simulink model "GUAM"  (R2024a)
settings: Solver=FixedStepAuto  StartTime=0.0  StopTime=SimIn.stopTime  FixedStep=0.01  RelTol=1e-6
InitFcn:
  | S = 0;
values from neighbouring files (symbols this model uses):
  SimIn = setup(SimIn, target)    [simSetup.m]
undefined symbols (not defined in the file or in its folder): SimPar
libraries: simulink x6, eeGeneralControl x5, dspstat3 x5, aerolibfltsims x2, dspnetwork x2
settings Model: SnapshotBufferSize=20  SnapshotInterval=1  PacingRate=0.100000  Creator=tbritton  LastModifiedBy=azmol
settings SolverCC: AlgebraicLoopSolver=TrustRegion  AutoInsertRateTranBlk=on  InsertRTBMode=Never (minimum delay)
settings DataIOCC: SaveFormat=StructureWithTime  SaveOutput=off  DSMLogging=off  SaveTime=off  ReturnWorkspaceOutputs=off
settings OptimizationCC: ReuseModelBlockBuffer=off
settings DebuggingCC: ReadBeforeWriteMsg=DisableAll  WriteAfterWriteMsg=DisableAll  WriteAfterReadMsg=DisableAll  UnconnectedInputMsg=warning  UnconnectedOutputMsg=warning  UnconnectedLineMsg=warning  InitInArrayFormatMsg=none
settings ModelReferenceCC: UpdateModelReferenceTargets=IfOutOfDate  EnableRefExpFcnMdlSchedulingChecks=on
settings SFSimCC: SFSimEcho=off  CustomCodeUndefinedFunction=UseInterfaceOnly
settings RTWCC: GPUComputeCapability=3.5  DLArmComputeVersion=19.05

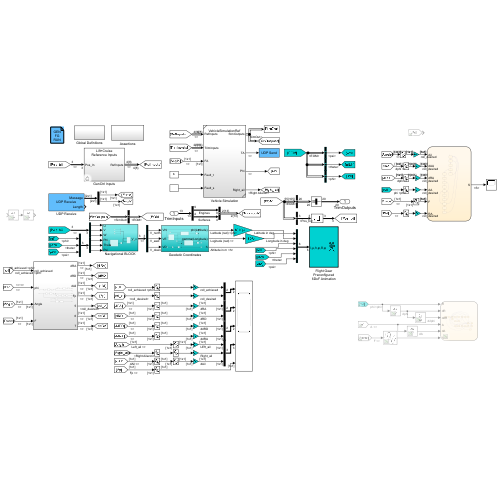
[thumbnail: Simulink's stored preview of the top-level diagram]
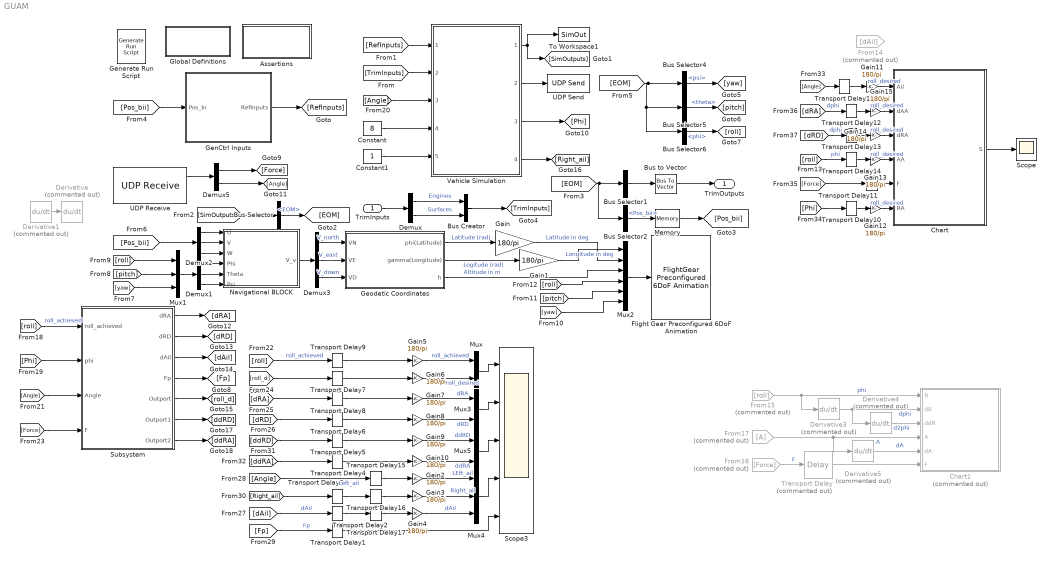
== system GUAM ==
  TrimInputs : Inport
  Assertions : Subsystem
  Bus Creator : BusCreator  Inputs=2  OutDataTypeStr=Bus: BUS_TRIM_INPUT
  Bus Selector : BusSelector  OutputSignals=Vehicle.EOM
  Bus Selector1 : BusSelector  OutputSignals=AirRelativeData.Veas,AirRelativeData.Vtot,AirRelativeData.alpha,AirRelativeData.beta,WorldRelativeData.gamma,WorldRelativeData.chi,InertialData.Asensed_bIb,AirRelativeData.Vtotdot,AirRelativeData.alphadot,AirRelativeData.betadot,WorldRelativeData.gammadot,WorldRelativeData.chidot,WorldRelativeData.VelDtH_bEh,WorldRelativeData.Euler.phi,WorldRelativeData.Euler.theta,WorldRelativeData.Euler.psi  OutputAsBus=on
  Bus Selector2 : BusSelector  OutputSignals=InertialData.Pos_bii
  Bus Selector4 : BusSelector  OutputSignals=WorldRelativeData.Euler.psi
  Bus Selector5 : BusSelector  OutputSignals=WorldRelativeData.Euler.theta
  Bus Selector6 : BusSelector  OutputSignals=WorldRelativeData.Euler.phi
  Bus to Vector : BusToVector
  Chart : Stateflow chart  TreatAsAtomicUnit=on
  Chart1 : Stateflow chart  Commented=on  TreatAsAtomicUnit=on
      settings: PortSchema="{\"entries\":[{\"content\":{\"sides\":[{\"content\":{\"connectorIds\":[\"In6\",\"In3\",\"In2\",\"In4\",\"In1\",\"In5\"]},\"type\":\"ConnectorPlacement.EquallySpacedRectSide\",\"uuid\":\"2c3cc659-f24d-4f43-a956-b726e491f665\"},{\"content\":{\"side\":\"RIGHT\"},\"type\":\"ConnectorPlacement.EquallySpacedRectSide\",\"uuid\":\"d5ffd018-8575-4a45-b274-c52cea02283c\"},{\"content\":{\"side\":\"TOP\"},\"type\":\"ConnectorPlacement.EquallySpacedRectSide\",\"uuid\":\"e163f1a1-9c0c-475f-9ea7-59fb8c09f8a6\"}]},\"type\":\"ConnectorPlacement.EquallySpacedConnector\",\"uuid\":\"e013bf2e-a49f-4647-8efb-e6a80c4823c8\"}],\"packageUris\":[\"http://schema.mathworks.com/mf0/Connector/R2020b\"],\"version\":\"1.0\"}"
  Constant : Constant  Value=8
  Constant1 : Constant
  Demux : Demux  Outputs=[SimIn.Trim.numEngines SimIn.Trim.numSurfaces]
  Demux1 : Demux  Outputs=3
  Demux2 : Demux  Outputs=3
  Demux3 : Demux  Outputs=3
  Demux5 : Demux  Outputs=2
  Derivative{,1,3..5} (5 alike) : Derivative  Commented=on
  Flight Gear Preconfigured 6DoF Animation : aerolibfltsims/FlightGear Preconfigured 6DoF Animation  xFlightGearVersion=v2019.1  DestinationIpAddress=127.0.0.1  DestinationPort=5502  SampleTime=1/100  packetVersion=24
  From14 : From  Commented=on  GotoTag=dAil
  From15 : From  Commented=on  GotoTag=roll
  From16 : From  Commented=on  GotoTag=Force
  From17 : From  Commented=on
  Gain{,1..15} (16 alike) : Gain  Gain=180/pi
  GenCtrl Inputs : Subsystem  Variant=on  VariantControl=Variant1
  Generate Run Script : aerolibfltsims/Generate Run Script  Architecture=Default  dataFlow=Send  GeometryModelName=c172p  AirportId=KSFO  RunwayId=10L  InitialAltitude=7224  InitialHeading=113  OffsetDistance=4.72  OffsetAzimuth=0  InstallScenery=off  DisableShaders=on  OriginAddress=127.0.0.1  DestinationPort=5502  OriginPort=5505  LocalAddress=127.0.0.1  OutputFileName=runfg.bat  FlightGearBaseDirectory=C:\guam_release_1p0_limited
  Geodetic Coordinates : Subsystem
  Global Definitions : Subsystem
  Memory : Memory
  Mux : Mux  Inputs=2
  Mux1 : Mux  Inputs=3
  Mux2 : Mux  Inputs=6
  Mux3 : Mux  Inputs=2
  Mux4 : Mux  Inputs=3
  Mux5 : Mux  Inputs=2
  Navigational BLOCK : Subsystem
  Scope : Scope
  Scope3 : Scope  NumInputPorts=5
  Subsystem : Subsystem
  To Workspace1 : ToWorkspace  VariableName=SimOut  SaveFormat=Timeseries  SampleTime=-1
      settings: Save2DSignal=2-D array (concatenate along first dimension)
  Transport Delay : TransportDelay  Commented=on  DelayTime=0.3
  Transport Delay{1..5,7..12,14} (12 alike) : TransportDelay  DelayTime=0.35
  Transport Delay13 : TransportDelay  DelayTime=0.81
  Transport Delay{15..18} (4 alike) : TransportDelay  DelayTime=0.3
  Transport Delay6 : TransportDelay  DelayTime=0.31
  UDP Receive : dspnetwork/UDP Receive  localURL='0.0.0.0'  localPort=25000  remoteURL='0.0.0.0'  remotePort=-1  recvBufferSize=8192  dims=2  signalDatatype=double  isComplex=off  isVarSize=off  showBlockingTime=off  blockingTime=0  sampletime=0.01  blockPlatform=[]
      settings: LibrarySourceBlock=dspsrcs4/UDP Receive
  UDP Send : dspnetwork/UDP Send  remoteURL='127.0.0.1'  remotePort=25001  localURL='0.0.0.0'  localPortSource=Automatically determine  localPort=-1  sendBufferSize=8192  sampletime=-1  blockPlatform=[]  separateLengthPort=0
      settings: LibrarySourceBlock=dspsnks4/UDP Send
  Vehicle Simulation : Subsystem  ReferencedSubsystem=VehicleSimulationRef
  TrimOutputs : Outport  OutDataTypeStr=double  VectorParamsAs1DForOutWhenUnconnected=off
  wires:
  TrimInputs/1 -> Demux/1
  Bus to Vector/1 -> TrimOutputs/1
  Bus Selector1/1 -> Bus to Vector/1
  GenCtrl Inputs/1(RefInputs) -> [RefInputs]
  Vehicle Simulation/1 -> To Workspace1/1, [SimOutputs]
  [TrimInputs] -> Vehicle Simulation/2
  [RefInputs] -> Vehicle Simulation/1
  [SimOutputs] -> Bus Selector/1
  Bus Selector/1 -> [EOM]  "<EOM>"
  Bus Creator/1 -> [TrimInputs]
  Demux/2 -> Bus Creator/2  "Surfaces"
  Demux/1 -> Bus Creator/1  "Engines"
  Bus Selector2/1 -> Memory/1  "<Pos_bii>"
  [EOM] -> Bus Selector2/1, Bus Selector1/1
  [Pos_bii] -> GenCtrl Inputs/1(Pos_In)
  Memory/1 -> [Pos_bii]
  Navigational BLOCK/1(V_v) -> Demux3/1
  Demux3/1 -> Geodetic Coordinates/1(VN)  "V_north"
  [EOM] -> Bus Selector6/1, Bus Selector5/1, Bus Selector4/1
  Bus Selector6/1 -> [roll]  "<phi>"
  Bus Selector5/1 -> [pitch]  "<theta>"
  Bus Selector4/1 -> [yaw]  "<psi>"
  [Pos_bii] -> Demux2/1
  Demux2/1 -> Navigational BLOCK/1(U)
  Demux2/2 -> Navigational BLOCK/2(V)
  Demux2/3 -> Navigational BLOCK/3(W)
  [pitch] -> Mux1/2
  [roll] -> Mux1/1
  [yaw] -> Mux1/3
  Mux1/1 -> Demux1/1
  Demux1/1 -> Navigational BLOCK/4(Phi)
  Demux1/2 -> Navigational BLOCK/5(Theta)
  Demux1/3 -> Navigational BLOCK/6(Psi)
  Demux3/2 -> Geodetic Coordinates/2(VE)  "V_east"
  Demux3/3 -> Geodetic Coordinates/3(VD)  "V_down"
  Geodetic Coordinates/1(phi(Latitude)) -> Gain/1  "Latitude (rad)"
  Gain/1 -> Mux2/2  "Latitude in deg"
  Geodetic Coordinates/2(gamma(Longitude)) -> Gain1/1  "Logitude (rad)"
  Gain1/1 -> Mux2/1  "Longitude in deg"
  Geodetic Coordinates/3(h) -> Mux2/3  "Altitude in m"
  [roll] -> Mux2/4
  [pitch] -> Mux2/5
  [yaw] -> Mux2/6
  Mux2/1 -> Flight Gear Preconfigured 6DoF Animation/1
  [roll] -> Transport Delay14/1  "phi"
  From15/1 -> Chart1/6(R), Derivative3/1  "phi"
  Derivative3/1 -> Chart1/3(dR), Derivative4/1  "dphi"
  Derivative4/1 -> Chart1/2(ddR)  "d2phi"
  From16/1 -> Transport Delay/1  "F"
  From17/1 -> Derivative5/1, Chart1/4(A)  "A"
  Derivative5/1 -> Chart1/1(dA)  "dA"
  Transport Delay/1 -> Chart1/5(F)
  Vehicle Simulation/3 -> [Phi]
  Constant/1 -> Vehicle Simulation/4
  Constant1/1 -> Vehicle Simulation/5
  Mux/1 -> Scope3/1
  Mux3/1 -> Scope3/2
  Vehicle Simulation/2 -> UDP Send/1
  UDP Receive/1 -> Demux5/1
  Demux5/1 -> [Force]
  Demux5/2 -> [Angle]
  [Angle] -> Vehicle Simulation/3
  [roll] -> Transport Delay9/1  "roll_achieved"
  [roll] -> Subsystem/1(roll_achieved)  "roll_achieved"
  [Phi] -> Subsystem/2(phi)
  [Angle] -> Subsystem/3(Angle)
  [Force] -> Subsystem/4(F)
  Subsystem/1(dRA) -> [dRA]
  Subsystem/2(dRD) -> [dRD]
  Subsystem/3(dAil) -> [dAil]
  Subsystem/4(Fp) -> [Fp]
  Subsystem/5(Outport) -> [roll_d]
  [roll_d] -> Transport Delay7/1
  [dRA] -> Transport Delay8/1
  [dRD] -> Transport Delay6/1
  [Angle] -> Transport Delay15/1  "Left_ail"
  [dAil] -> Transport Delay2/1  "dAil"
  Mux4/1 -> Scope3/4
  [Fp] -> Transport Delay1/1  "Fp"
  Vehicle Simulation/4 -> [Right_ail]
  [Right_ail] -> Transport Delay3/1
  Subsystem/6(Outport1) -> [ddRD]
  Subsystem/7(Outport2) -> [ddRA]
  [ddRA] -> Transport Delay4/1
  [ddRD] -> Transport Delay5/1
  Mux5/1 -> Scope3/3
  Gain2/1 -> Mux4/1  "LEft_ail"
  Gain3/1 -> Mux4/2  "Right_ail"
  Gain4/1 -> Mux4/3  "dAil"
  Gain5/1 -> Mux/1  "roll_achieved"
  Gain6/1 -> Mux/2  "roll_desired"
  Gain7/1 -> Mux3/1  "dRA"
  Gain8/1 -> Mux3/2  "dRD"
  Gain9/1 -> Mux5/1  "ddRD"
  Gain10/1 -> Mux5/2  "ddRA"
  Transport Delay3/1 -> Transport Delay16/1
  Derivative1/1 -> Derivative/1
  [dRA] -> Transport Delay12/1  "dphi"
  [Angle] -> Transport Delay18/1
  [Phi] -> Transport Delay10/1
  [dRD] -> Transport Delay13/1  "dphi"
  [Force] -> Transport Delay11/1
  Chart/1(S) -> Scope/1
  Transport Delay1/1 -> Scope3/5
  Transport Delay2/1 -> Transport Delay17/1
  Transport Delay4/1 -> Gain10/1
  Transport Delay5/1 -> Gain9/1
  Transport Delay6/1 -> Gain8/1
  Transport Delay8/1 -> Gain7/1
  Transport Delay7/1 -> Gain6/1
  Transport Delay9/1 -> Gain5/1
  Transport Delay12/1 -> Gain15/1
  Transport Delay13/1 -> Gain14/1
  Transport Delay14/1 -> Gain13/1
  Transport Delay10/1 -> Gain12/1
  Transport Delay11/1 -> Chart/5(F)
  Gain11/1 -> Chart/1(Ail)  "roll_desired"
  Gain12/1 -> Chart/6(RA)  "roll_desired"
  Gain13/1 -> Chart/4(AA)  "roll_desired"
  Gain14/1 -> Chart/3(dRA)  "roll_desired"
  Gain15/1 -> Chart/2(dAA)  "roll_desired"
  Transport Delay15/1 -> Gain2/1
  Transport Delay16/1 -> Gain3/1
  Transport Delay17/1 -> Gain4/1
  Transport Delay18/1 -> Gain11/1

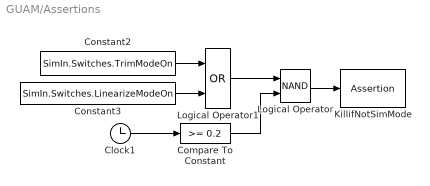
== system GUAM/Assertions ==
  Clock1 : Clock
  Compare To Constant : simulink/Logic and Bit Operations/Compare To Constant  relop=>=  const=0.2  OutDataTypeStr=boolean  ZeroCross=off
  Constant2 : Constant  Value=SimIn.Switches.TrimModeOn
  Constant3 : Constant  Value=SimIn.Switches.LinearizeModeOn
  KillifNotSimMode : Assertion  AssertionFailFcn="warndlg('Running simulation with TrimMode or LinearizeMode engaged.  Run setup.m to reset.','Warning!')"
  Logical Operator : Logic  Operator=NAND  AllPortsSameDT=off  OutDataTypeStr=boolean
  Logical Operator1 : Logic  Operator=OR  AllPortsSameDT=off  OutDataTypeStr=boolean
  wires:
  Constant2/1 -> Logical Operator1/1
  Compare To Constant/1 -> Logical Operator/2
  Clock1/1 -> Compare To Constant/1
  Logical Operator/1 -> KillifNotSimMode/1
  Constant3/1 -> Logical Operator1/2
  Logical Operator1/1 -> Logical Operator/1

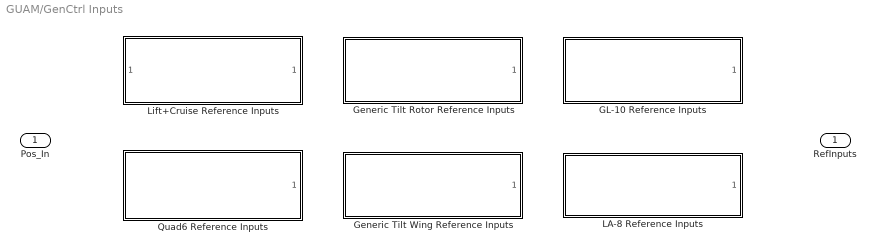
== system GUAM/GenCtrl Inputs ==
  Pos_In : Inport
  GL-10 Reference Inputs : Subsystem  VariantControl=GVS_VEH_TYPE_GL10  ReferencedSubsystem=GL_10_Reference_Inputs
  Generic Tilt Rotor Reference Inputs : Subsystem  VariantControl=GVS_VEH_TYPE_GTR  ReferencedSubsystem=GTR_Reference_Inputs
  Generic Tilt Wing Reference Inputs : Subsystem  VariantControl=GVS_VEH_TYPE_GTW  ReferencedSubsystem=GTW_Reference_Inputs
  LA-8 Reference Inputs : Subsystem  VariantControl=GVS_VEH_TYPE_LA8  ReferencedSubsystem=LA_8_Reference_Inputs
  Lift+Cruise Reference Inputs : Subsystem  VariantControl=GVS_VEH_TYPE_LC  ReferencedSubsystem=Lift_Cruise_Reference_Inputs
  Quad6 Reference Inputs : Subsystem  VariantControl=GVS_VEH_TYPE_QUAD6  ReferencedSubsystem=Quad6_Reference_Inputs
  RefInputs : Outport  OutDataTypeStr=Bus: BUS_REF_INPUT

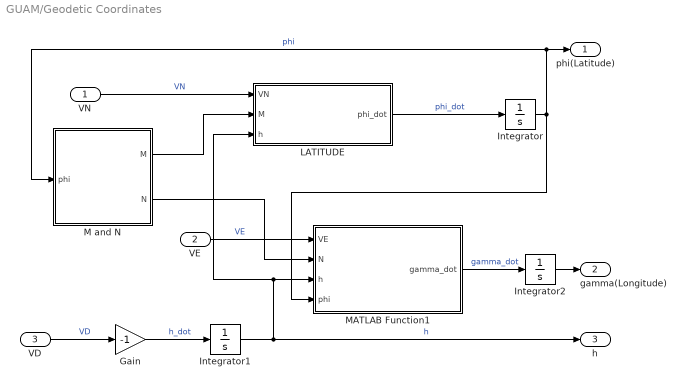
== system GUAM/Geodetic Coordinates ==
  VN : Inport
  VE : Inport  Port=2
  VD : Inport  Port=3
  Gain : Gain  Gain=-1
  Integrator : Integrator
  Integrator1 : Integrator
  Integrator2 : Integrator
  LATITUDE : MATLAB Function  TreatAsAtomicUnit=on
  M and N : Subsystem
  MATLAB Function1 : MATLAB Function  TreatAsAtomicUnit=on
  phi(Latitude) : Outport
  gamma(Longitude) : Outport  Port=2
  h : Outport  Port=3
  wires:
  VN/1 -> LATITUDE/1(VN)  "VN"
  M and N/1(M) -> LATITUDE/2(M)
  VE/1 -> MATLAB Function1/1(VE)  "VE"
  Integrator/1 -> M and N/1(phi), phi(Latitude)/1, MATLAB Function1/4(phi)  "phi"
  LATITUDE/1(phi_dot) -> Integrator/1  "phi_dot"
  M and N/2(N) -> MATLAB Function1/2(N)
  VD/1 -> Gain/1  "VD"
  Gain/1 -> Integrator1/1  "h_dot"
  Integrator1/1 -> LATITUDE/3(h), MATLAB Function1/3(h), h/1  "h"
  MATLAB Function1/1(gamma_dot) -> Integrator2/1  "gamma_dot"
  Integrator2/1 -> gamma(Longitude)/1

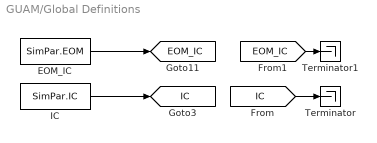
== system GUAM/Global Definitions ==
  EOM_IC : Constant  Value=SimPar.EOM  OutDataTypeStr=Bus: BUS_PARAM_EOM
  IC : Constant  Value=SimPar.IC  OutDataTypeStr=Bus: BUS_PARAM_IC
  Terminator : Terminator
  Terminator1 : Terminator
  tag scope: EOM_IC=global, IC=global
  wires:
  IC/1 -> [IC]
  EOM_IC/1 -> [EOM_IC]
  [IC] -> Terminator/1
  [EOM_IC] -> Terminator1/1

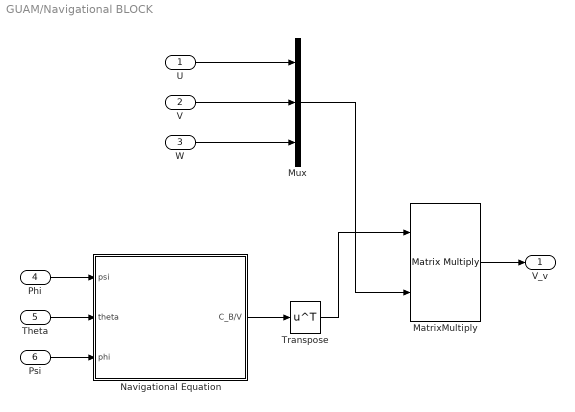
== system GUAM/Navigational BLOCK ==
  U : Inport
  V : Inport  Port=2
  W : Inport  Port=3
  Phi : Inport  Port=4
  Theta : Inport  Port=5
  Psi : Inport  Port=6
  MatrixMultiply : Product  Multiplication=Matrix(*)
  Mux : Mux  Inputs=3
  Navigational Equation : Subsystem
  Transpose : Math  Operator=transpose
  V_v : Outport
  wires:
  Phi/1 -> Navigational Equation/1(psi)
  Theta/1 -> Navigational Equation/2(theta)
  Psi/1 -> Navigational Equation/3(phi)
  V/1 -> Mux/2
  U/1 -> Mux/1
  W/1 -> Mux/3
  MatrixMultiply/1 -> V_v/1
  Mux/1 -> MatrixMultiply/2
  Navigational Equation/1(C_B/V) -> Transpose/1
  Transpose/1 -> MatrixMultiply/1

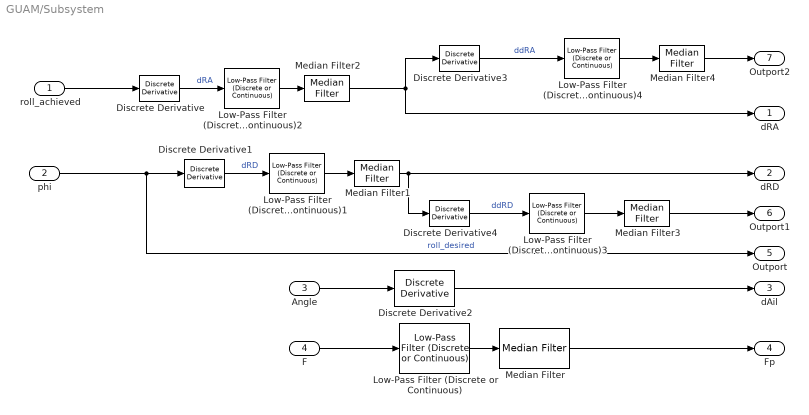
== system GUAM/Subsystem ==
  roll_achieved : Inport
  phi : Inport  Port=2
  Angle : Inport  Port=3
  F : Inport  Port=4
  Discrete Derivative{,1..4} (5 alike) : simulink/Discrete/Discrete Derivative  gainval=1.0  ICPrevScaledInput=0.0  OutMin=[]  OutMax=[]  OutDataType=fixdt(1, 16)  OutScaling=2^-10  DoSatur=off
  Low-Pass Filter (Discrete or Continuous){,1..4} (5 alike) : eeGeneralControl/Low-Pass Filter (Discrete or Continuous)  K=1  T=0.05  B=inf  A=-inf  init_option=Inherited from block input  x0=0  Ts=-1
  Median Filter{,1..4} (5 alike) : dspstat3/Median Filter  WindowLength=5  SimulateUsing=Interpreted execution
      settings: LibrarySourceBlock=|
      | dspfdesign/Median
      | Filter
  dRA : Outport
  dRD : Outport  Port=2
  dAil : Outport  Port=3
  Fp : Outport  Port=4
  Outport : Outport  Port=5
  Outport1 : Outport  Port=6
  Outport2 : Outport  Port=7
  wires:
  Median Filter/1 -> Fp/1
  phi/1 -> Discrete Derivative1/1, Outport/1  "roll_desired"
  Low-Pass Filter (Discrete or Continuous)/1 -> Median Filter/1
  Discrete Derivative2/1 -> dAil/1
  roll_achieved/1 -> Discrete Derivative/1
  F/1 -> Low-Pass Filter (Discrete or Continuous)/1
  Angle/1 -> Discrete Derivative2/1
  Discrete Derivative1/1 -> Low-Pass Filter (Discrete or Continuous)1/1  "dRD"
  Discrete Derivative/1 -> Low-Pass Filter (Discrete or Continuous)2/1  "dRA"
  Discrete Derivative3/1 -> Low-Pass Filter (Discrete or Continuous)4/1  "ddRA"
  Discrete Derivative4/1 -> Low-Pass Filter (Discrete or Continuous)3/1  "ddRD"
  Low-Pass Filter (Discrete or Continuous)1/1 -> Median Filter1/1
  Median Filter1/1 -> dRD/1, Discrete Derivative4/1
  Low-Pass Filter (Discrete or Continuous)2/1 -> Median Filter2/1
  Median Filter2/1 -> dRA/1, Discrete Derivative3/1
  Low-Pass Filter (Discrete or Continuous)3/1 -> Median Filter3/1
  Median Filter3/1 -> Outport1/1
  Low-Pass Filter (Discrete or Continuous)4/1 -> Median Filter4/1
  Median Filter4/1 -> Outport2/1

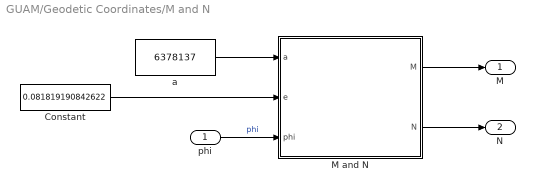
== system GUAM/Geodetic Coordinates/M and N ==
  phi : Inport
  Constant : Constant  Value=0.081819190842622
  M and N : MATLAB Function  TreatAsAtomicUnit=on
  a : Constant  Value=6378137
  M : Outport
  N : Outport  Port=2
  wires:
  phi/1 -> M and N/3(phi)  "phi"
  M and N/1(M) -> M/1
  a/1 -> M and N/1(a)
  Constant/1 -> M and N/2(e)
  M and N/2(N) -> N/1

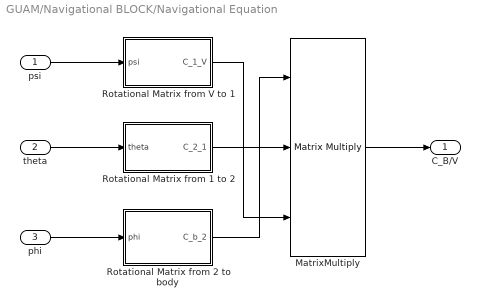
== system GUAM/Navigational BLOCK/Navigational Equation ==
  psi : Inport
  theta : Inport  Port=2
  phi : Inport  Port=3
  MatrixMultiply : Product  Inputs=3  Multiplication=Matrix(*)
  Rotational Matrix from 1 to 2 : MATLAB Function  TreatAsAtomicUnit=on
  Rotational Matrix from 2 to body : MATLAB Function  TreatAsAtomicUnit=on
  Rotational Matrix from V to 1 : MATLAB Function  TreatAsAtomicUnit=on
  C_B/V : Outport
  wires:
  psi/1 -> Rotational Matrix from V to 1/1(psi)
  theta/1 -> Rotational Matrix from 1 to 2/1(theta)
  phi/1 -> Rotational Matrix from 2 to body/1(phi)
  MatrixMultiply/1 -> C_B/V/1
  Rotational Matrix from 2 to body/1(C_b_2) -> MatrixMultiply/1
  Rotational Matrix from V to 1/1(C_1_V) -> MatrixMultiply/3
  Rotational Matrix from 1 to 2/1(C_2_1) -> MatrixMultiply/2

== stateflow chart GUAM/Chart1 ==
  state constant_angle
  state s1
  state s2
  state s3
  state s4
  state s9
  state s10
  state s11
  state s19
  state s20
  state s23
  state s12
  state s22
  state s17
  state s16
  state s15
  state s14
  state s13
  state s24
  state s25
  s11 -> s2 [order 3] : [dR>0.01 && ddR>0.01]
  s10 -> s2 [order 3] : [dR>0.01 && ddR>0.01]
  s2 -> s9 [order 2] : [dR>0.01 && ddR<-0.01]
  s11 -> s9 [order 2] : [dR>0.01 && ddR<-0.01]
  s4 -> s2 [order 2] : [dR>0.01 && ddR>0.01]
  (default) -> constant_angle
  s1 -> s2 : [dR>0/01 && ddR>0.01]
  s17 -> s2 [order 3] : [dR>0.01 && ddR>0.01]
  constant_angle -> s1 : [R > 0]
  s2 -> s3 [order 1] : [F>0.01]
  s3 -> s4 [order 1] : [A<-1]
  s4 -> s9 [order 1] : [dR>0.01 && ddR<-0.01]
  s9 -> s10 [order 1] : [F<-0.01]
  s10 -> s11 [order 1] : [A>1]
  s16 -> s2 [order 3] : [dR>0.01 && ddR>0.01]
  s15 -> s2 [order 2] : [dR>0.01 && ddR>0.01]
  s14 -> constant_angle [order 3] : [R == 0]
  s2 -> s19 [order 3] : [F<-0.01]
  s3 -> s9 [order 2] : [dR>0.01 && ddR<-0.01]
  s23 -> s9 [order 2] : [dR>0.01 && ddR<-0.01]
  s9 -> s12 [order 2] : [dR<-0.01 && ddR<-0.01]
  s10 -> s12 [order 2] : [dR<-0.01 && ddR<-0.01]
  s11 -> s12 [order 1] : [dR<-0.01 && ddR<-0.01]
  s23 -> s19 [order 1] : [dR>0.01 && ddR>0.01]
  s19 -> s20 : [F<-0.01]
  s20 -> s23 : [dA>-1 && dA<1]
  s12 -> s22 [order 3] : [F>0.01]
  s17 -> s12 [order 1] : [dR<-0.01 && ddR<-0.01]
  s16 -> s12 [order 2] : [dR<-0.01 && ddR<-0.01]
  s14 -> s12 [order 2] : [dR<-0.01 && ddR<-0.01]
  s12 -> s15 [order 1] : [dR<-0.01 && ddR>0.01]
  s13 -> s15 [order 2] : [dR<-0.01 && ddR>0.01]
  s12 -> s13 [order 2] : [F<-0.01]
  s25 -> s22 [order 1] : [dR<-0.01 && ddR<-0.01]
  s22 -> s24 : [F>0.01]
  s16 -> s17 [order 1] : [A < -1 ]
  s15 -> s16 [order 1] : [F>0.01]
  s14 -> s15 [order 1] : [dR<-0.01 && ddR>0.01]
  s13 -> s14 [order 1] : [A>1]
  s17 -> s15 [order 2] : [dR<-0.01 && ddR>0.01]
  s25 -> s15 [order 2] : [dR<-0.01 && ddR>0.01]
  s24 -> s25 : [dA>-1 && dA<1]
  data: dA input; ddR input; dR input; A input; F input; R input

== stateflow chart GUAM/Chart ==
  state s1
  state s2
  state s20
  state s3
  state s21
  state s4
  state s22
  state s5
    if k ~=0
    S =k;
    end
  state s23
  state s10
  state s24
  state s11
  state s25
  state s42
  state s12
  state s26
  state s34
  state s13
  state s27
  state s35
  state s14
  state s28
  state s36
  state s15
  state s29
  state s37
  state s16
  state s17
  state s30
  state s38
  state s18
  state s31
  state s39
  state s19
    S = 1;
    k = -1;
  state s322
  state s40
  state s33
    S = 0;
    k = 1;
  state s41
    S = 0;
    k = 1;
  (default) -> s1 : {k = 0}
  s5 -> s1 : [-5e-2<dRA && dRA<5e-2]
  s19 -> s1 : [-5e-2<dRA && dRA<5e-2]
  s1 -> s20 [order 2] : [RA>0.5]
  s1 -> s2 [order 1] : [-0.5<RA && RA<0.5 ]
  s2 -> s17 [order 2] : [F > 5]
  s2 -> (junction 25) [order 1]
  s20 -> s21 : [F>5]
  s33 -> (junction 25) [order 1]
  (junction 25) -> s3 : after (0.01,sec)[(k == 0) && (-5<F && F<5)]
  s23 -> s21 [order 2] : [F>5]
  s3 -> s4 : [-0.1<Ail && Ail<0.1]
  s21 -> s22 : [Ail < 0.1 ]
  s4 -> s10 [order 2] : [dAA < -9e-3]
  s4 -> s5 [order 1] : after (0.01,sec)[-0.3<AA && AA <0.3]
  s22 -> s23 : [dAA > 9e-3]
  s25 -> s23 [order 2] : [dAA > 9e-3]
  s23 -> s24 [order 1] : [ F < -2]
  s10 -> s11 : [dRA > 5e-2]
  s24 -> s25 : [Ail > 0.1]
  s11 -> s12 : [F > 5 ]
  s14 -> s12 [order 2] : after(0.04, sec)[F > 5]
  s25 -> (junction 135) [order 3]
  (junction 135) -> s42 : [F > 5]
  s41 -> (junction 135) [order 1]
  s25 -> s26 [order 1] : [-5<F && F<5]
  s34 -> s42 [order 1] : [-5e-2<dRA && dRA<5e-2]
  s42 -> s34 : [Ail < -0.1]
  s12 -> s13 : [Ail <-0.1]
  s27 -> s26 [order 2] : [-5e-2<dRA && dRA<5e-2]
  s26 -> s27 : [-0.1<Ail && Ail<0.1]
  s34 -> s35 [order 2] : [dAA < -9e-3]
  s13 -> s14 : after (0.02, sec) [ dAA > 9e-3 ]
  s16 -> s14 [order 2] : [ dAA > 9e-3 ]
  s14 -> s17 [order 3] : after(0.01, sec)[F > 5]
  s27 -> s28 [order 1] : [RA < -0.5]
  s35 -> s36 : [RA>0.5]
  s14 -> s15 [order 1] : [F < -2]
  s28 -> s29 : [F < -5]
  s36 -> s37 : [F > 5]
  s15 -> s16 : [Ail < -0.1]
  s31 -> s29 [order 2] : [F < -5]
  s39 -> s37 [order 1] : [F > 5]
  s29 -> s30 : [Ail > 0.1]
  s37 -> s38 : [Ail < -0.1]
  s16 -> s17 [order 1] : [F > 5]
  s17 -> s18 : [Ail < -0.1]
  s30 -> s31 : [dAA < -9e-3]
  s38 -> s39 : [dAA > 9e-3]
  s33 -> s31 [order 2] : [dAA < -9e-3]
  s41 -> s39 [order 2] : [dAA > 9e-3]
  s18 -> s19 : [-0.3<AA && AA <0.3]
  s31 -> s322 [order 1] : [F > 5]
  s39 -> s40 [order 2] : [F < -5]
  s322 -> s33 : [Ail < -0.1]
  s40 -> s41 : [Ail > 0.1]
  data: Ail input; dAA input; dRA input; AA input; F input; RA input; S output; k local

== matlab function GUAM/Geodetic Coordinates/M and N/M and N ==
  data: a input; M output; e input; phi input; N output
function[M,N]=M_N(a,e,phi)

M=(a*(1-e*2)/(1-(e^2)*sin(phi))^3/2);  % Meridian Radius of Curvature

N=a/(1-(e^2)*(sin(phi)^2))^3/2;        % Prime verical radius of curvature

end

== matlab function GUAM/Geodetic Coordinates/LATITUDE ==
  data: VN input; phi_dot output; M input; h input
function phi_dot =Latitude_Rate(VN,M,h)
% Calculating the Rate of change of Latitude

phi_dot=VN/(M+h);
end

== matlab function GUAM/Geodetic Coordinates/MATLAB Function1 ==
  data: VE input; gamma_dot output; N input; h input; phi input
function gamma_dot =Longitude_Rate(VE,N,h,phi)

% Calculating the Rate of change of the Longitude

gamma_dot=VE/((N+h)*cos(phi));
end

== matlab function GUAM/Navigational BLOCK/Navigational Equation/Rotational Matrix from V to 1 ==
  data: psi input; C_1_V output
function C_1_V = fcn(psi)

% Calculating the Rotaional Matrix  from the NED to 1 frame

C_1_V=[cos(psi) sin(psi) 0; -sin(psi) cos(psi) 0; 0 0 1];

end

== matlab function GUAM/Navigational BLOCK/Navigational Equation/Rotational Matrix from 1 to 2 ==
  data: theta input; C_2_1 output
function C_2_1 = fcn(theta)

% Roational Matrix From the 1 frame to 2 frame

C_2_1=[cos(theta) 0 -sin(theta); 0 1 0; sin(theta) 0 cos(theta)];

end

== matlab function GUAM/Navigational BLOCK/Navigational Equation/Rotational Matrix from 2 to body ==
  data: phi input; C_b_2 output
function C_b_2 = fcn(phi)

% Roational Matrix from the 2 frame to body frame
C_b_2=[1 0 0; 0 cos(phi) sin(phi); 0 -sin(phi) cos(phi)];
end
